simulink model "HRXDUAL_Delay"  (R2023b)
settings: Solver=FixedStepDiscrete  StartTime=0.0  StopTime=Inf  FixedStep=0.0001  RelTol=1e-3  EnableMultiTasking=on
libraries: canmsglib x24, c280xlib x24, simulink x11
(part 1 of 2)
settings Model: SimulationMode=external  ExtModeTrigDuration=8  Creator=eisaa  LastModifiedBy=pc_ha
settings SolverCC: AlgebraicLoopSolver=TrustRegion
settings OptimizationCC: DefaultUnderspecifiedDataType=single  EnhancedBackFolding=on  PassReuseOutputArgsAs=Individual arguments  MaxStackSize=1024  OptimizeBlockOrder=speed  DifferentSizesBufferReuse=on  OptimizationCustomize=off  DenormalBehavior=FlushToZero  EfficientTunableParamExpr=on
settings DebuggingCC: ParameterTunabilityLossMsg=error  UnconnectedInputMsg=warning  UnconnectedOutputMsg=warning  UnconnectedLineMsg=warning
settings HardwareCC: ProdBitPerChar=16  ProdBitPerInt=16  ProdBitPerPointer=32  ProdBitPerSizeT=32  ProdBitPerPtrDiffT=32  ProdLargestAtomicInteger=Integer  ProdLargestAtomicFloat=None  ProdWordSize=16  ProdLongLongMode=on  ProdHWDeviceType=Texas Instruments->C2000
settings ModelReferenceCC: EnableRefExpFcnMdlSchedulingChecks=on
settings SFSimCC: MATLABDynamicMemAlloc=off
settings RTWCC: Description=Embedded Coder  SystemTargetFile=ert.tlc  HardwareBoard=TI Piccolo F28069M LaunchPad  TemplateMakefile=ert_default_tmf  Toolchain=Texas Instruments Code Composer Studio (C2000)  CodeProfilingSaveOptions=AllData  DLArmComputeVersion=19.05
settings CodeAppCC: ForceParamTrailComments=on  IgnoreCustomStorageClasses=off  OperatorAnnotations=on  SimulinkDataObjDesc=on  SFDataObjDesc=on  InsertBlockDesc=on
settings ERTTargetCC: CodeReplacementLibrary=TI C28x  SupportContinuousTime=on  ExtModeTransport=4  ExtModeStaticAlloc=on  ExtModeAutomaticAllocSize=off  ExtModeStaticAllocSize=10000  ExtModeMexFile=ext_xcp  ExtModeMexArgs='127.0.0.1' 0 17725  ExtModeIntrfLevel=Level2 - Open

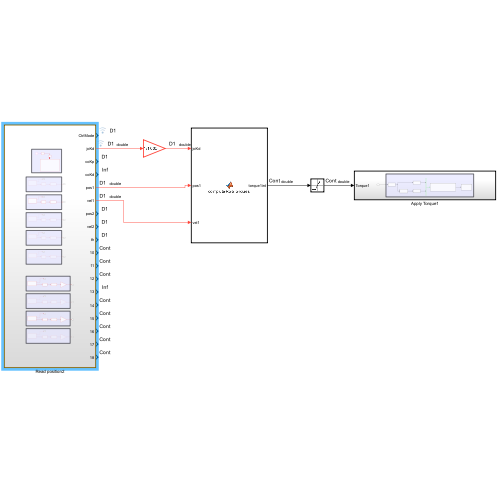
[thumbnail: Simulink's stored preview of the top-level diagram]
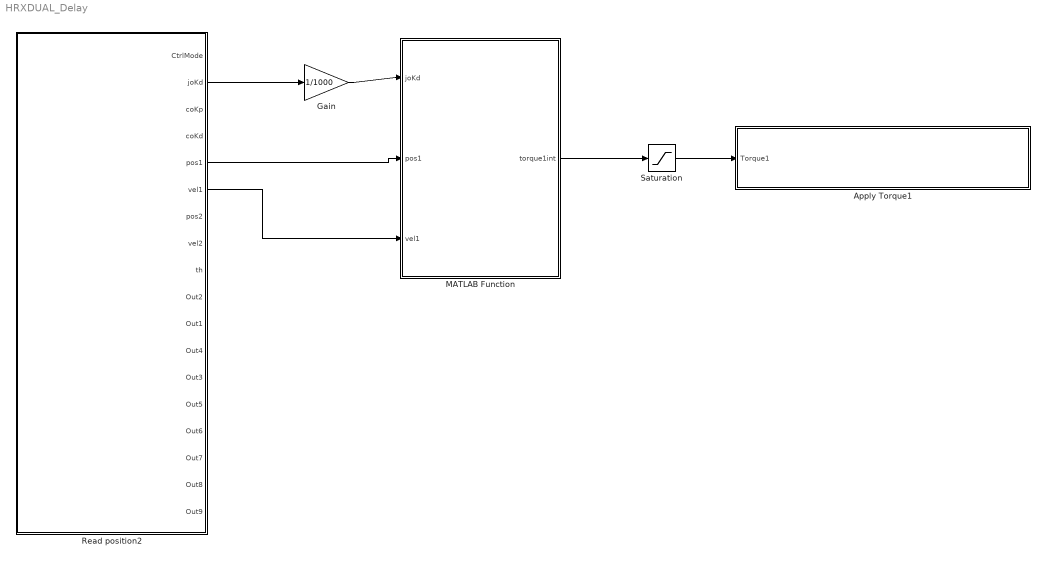
== system HRXDUAL_Delay ==
  Apply Torque1 : Subsystem
  Gain : Gain  Gain=1/1000
  MATLAB Function : MATLAB Function  TreatAsAtomicUnit=on
  Read position2 : Subsystem
  Saturation : Saturate  UpperLimit=1750  LowerLimit=-1750
  wires:
  Read position2/2(joKd) -> Gain/1
  Gain/1 -> MATLAB Function/1(joKd)
  Read position2/5(pos1) -> MATLAB Function/2(pos1)
  Read position2/6(vel1) -> MATLAB Function/3(vel1)
  Saturation/1 -> Apply Torque1/1(Torque1)
  MATLAB Function/1(torque1int) -> Saturation/1

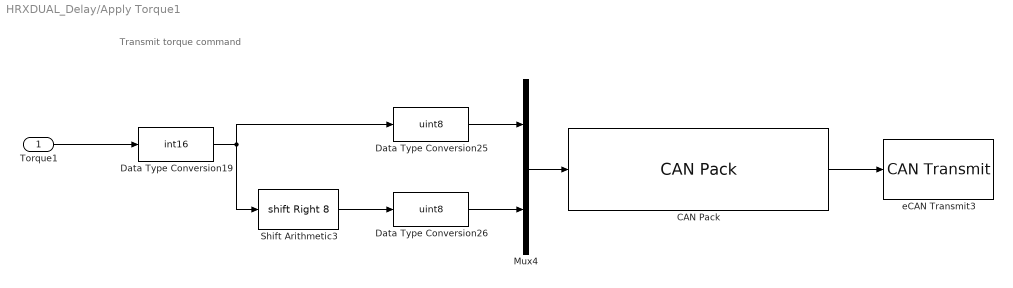
== system HRXDUAL_Delay/Apply Torque1 ==
  note: Transmit torque command
  Torque1 : Inport
  CAN Pack : canmsglib/CAN Pack  MsgList=(none)  MsgName=CAN Msg  MsgIDType=Standard (11-bit identifier)  MsgIdentifier=hex2dec('0x301')  MsgLength=2  Remote=off  ApplyMinMax=off  BusOutput=off  SignalInfo={}
      settings: LibrarySourceBlock=c2000lib/Target Communication/CAN Pack  DataFormat=raw data
  Data Type Conversion19 : DataTypeConversion  OutDataTypeStr=int16  SaturateOnIntegerOverflow=off  RndMeth=Floor
  Data Type Conversion25 : DataTypeConversion  OutDataTypeStr=uint8  SaturateOnIntegerOverflow=off  RndMeth=Floor
  Data Type Conversion26 : DataTypeConversion  OutDataTypeStr=uint8  SaturateOnIntegerOverflow=off  RndMeth=Floor
  Mux4 : Mux  Inputs=2
  Shift Arithmetic3 : ArithShift  BitShiftNumber=8  BitShiftDirection=Right
  eCAN Transmit3 : c280xlib/CAN Transmit  chipFamily=C280x  useModule=CAN_A  mailboxNo=1  messageID=hex2dec('0x301')  messageType=Standard (11-bit identifier)  enableBlockingMode=on  postInterrupt=off  interruptLine=0
  wires:
  CAN Pack/1 -> eCAN Transmit3/1
  Data Type Conversion19/1 -> Data Type Conversion25/1, Shift Arithmetic3/1
  Mux4/1 -> CAN Pack/1
  Data Type Conversion26/1 -> Mux4/2
  Torque1/1 -> Data Type Conversion19/1
  Shift Arithmetic3/1 -> Data Type Conversion26/1
  Data Type Conversion25/1 -> Mux4/1

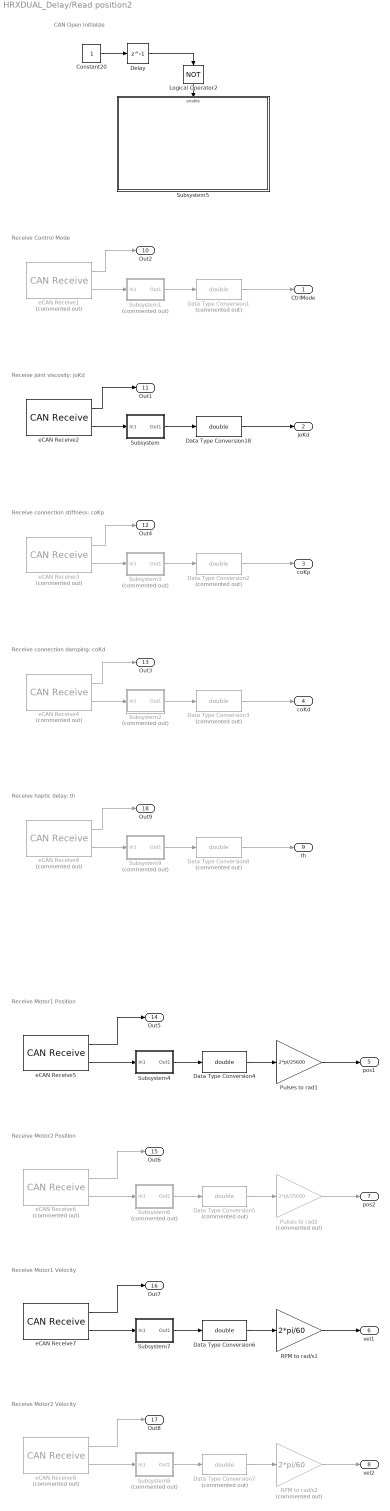
== system HRXDUAL_Delay/Read position2 ==
  note: CAN Open Initialize
  note: Receive Control Mode
  note: Receive joint viscosity: joKd
  note: Receive connection damping: coKd
  note: Receive connection stiffness: coKp
  note: Receive Motor1 Position
  note: Receive Motor2 Position
  note: Receive Motor2 Velocity
  note: Receive Motor1 Velocity
  note: Receive haptic delay: th
  Constant20 : Constant
  Data Type Conversion{1..3,5,7..8} (6 alike) : DataTypeConversion  Commented=on  OutDataTypeStr=double  SaturateOnIntegerOverflow=off  RndMeth=Floor
  Data Type Conversion18 : DataTypeConversion  OutDataTypeStr=double  SaturateOnIntegerOverflow=off  RndMeth=Floor
  Data Type Conversion4 : DataTypeConversion  OutDataTypeStr=double  SaturateOnIntegerOverflow=off  RndMeth=Floor
  Data Type Conversion6 : DataTypeConversion  OutDataTypeStr=double  SaturateOnIntegerOverflow=off  RndMeth=Floor
  Delay : Delay  DelayLength=1
  Logical Operator2 : Logic  Operator=NOT  AllPortsSameDT=off  OutDataTypeStr=boolean
  Pulses to rad1 : Gain  Gain=2*pi/25600
  Pulses to rad2 : Gain  Commented=on  Gain=2*pi/25600
  RPM to rad/s1 : Gain  Gain=2*pi/60
  RPM to rad/s2 : Gain  Commented=on  Gain=2*pi/60
  Subsystem : Subsystem
  Subsystem1 : Subsystem  Commented=on
  Subsystem2 : Subsystem  Commented=on
  Subsystem3 : Subsystem  Commented=on
  Subsystem4 : Subsystem
  Subsystem5 : Subsystem
  Subsystem6 : Subsystem  Commented=on
  Subsystem7 : Subsystem
  Subsystem8 : Subsystem  Commented=on
  Subsystem9 : Subsystem  Commented=on
  eCAN Receive1 : c280xlib/CAN Receive  Commented=on  chipFamily=C280x  useModule=CAN_A  mailboxNo=7  messageID=hex2dec('0x666')  messageType=Standard (11-bit identifier)  enableAcceptanceFiltering=off  messageIDMask=0  sampleTime=-1  dataType=CAN_MESSAGE_TYPE  outputAction=Output last received values  initValue=1  outputMessageID=off  outputMessageLength=off  outputMessageTimeStamp=off  postInterrupt=off  interruptLine=0
  eCAN Receive2 : c280xlib/CAN Receive  chipFamily=C280x  useModule=CAN_A  mailboxNo=8  messageID=hex2dec('0x667')  messageType=Standard (11-bit identifier)  enableAcceptanceFiltering=off  messageIDMask=0  sampleTime=-1  dataType=CAN_MESSAGE_TYPE  outputAction=Output last received values  initValue=0  outputMessageID=off  outputMessageLength=off  outputMessageTimeStamp=off  postInterrupt=off  interruptLine=0
  eCAN Receive3 : c280xlib/CAN Receive  Commented=on  chipFamily=C280x  useModule=CAN_A  mailboxNo=9  messageID=hex2dec('0x668')  messageType=Standard (11-bit identifier)  enableAcceptanceFiltering=off  messageIDMask=0  sampleTime=-1  dataType=CAN_MESSAGE_TYPE  outputAction=Output last received values  initValue=0  outputMessageID=off  outputMessageLength=off  outputMessageTimeStamp=off  postInterrupt=off  interruptLine=0
  eCAN Receive4 : c280xlib/CAN Receive  Commented=on  chipFamily=C280x  useModule=CAN_A  mailboxNo=10  messageID=hex2dec('0x669')  messageType=Standard (11-bit identifier)  enableAcceptanceFiltering=off  messageIDMask=0  sampleTime=-1  dataType=CAN_MESSAGE_TYPE  outputAction=Output last received values  initValue=0  outputMessageID=off  outputMessageLength=off  outputMessageTimeStamp=off  postInterrupt=off  interruptLine=0
  eCAN Receive5 : c280xlib/CAN Receive  chipFamily=C280x  useModule=CAN_A  mailboxNo=3  messageID=hex2dec('0x381')  messageType=Standard (11-bit identifier)  enableAcceptanceFiltering=off  messageIDMask=0  sampleTime=-1  dataType=CAN_MESSAGE_TYPE  outputAction=Output last received values  initValue=0  outputMessageID=off  outputMessageLength=off  outputMessageTimeStamp=off  postInterrupt=off  interruptLine=0
  eCAN Receive6 : c280xlib/CAN Receive  Commented=on  chipFamily=C280x  useModule=CAN_A  mailboxNo=4  messageID=hex2dec('0x382')  messageType=Standard (11-bit identifier)  enableAcceptanceFiltering=off  messageIDMask=0  sampleTime=-1  dataType=CAN_MESSAGE_TYPE  outputAction=Output last received values  initValue=0  outputMessageID=off  outputMessageLength=off  outputMessageTimeStamp=off  postInterrupt=off  interruptLine=0
  eCAN Receive7 : c280xlib/CAN Receive  chipFamily=C280x  useModule=CAN_A  mailboxNo=5  messageID=hex2dec('0x481')  messageType=Standard (11-bit identifier)  enableAcceptanceFiltering=off  messageIDMask=0  sampleTime=-1  dataType=CAN_MESSAGE_TYPE  outputAction=Output last received values  initValue=0  outputMessageID=off  outputMessageLength=off  outputMessageTimeStamp=off  postInterrupt=off  interruptLine=0
  eCAN Receive8 : c280xlib/CAN Receive  Commented=on  chipFamily=C280x  useModule=CAN_A  mailboxNo=6  messageID=hex2dec('0x482')  messageType=Standard (11-bit identifier)  enableAcceptanceFiltering=off  messageIDMask=0  sampleTime=-1  dataType=CAN_MESSAGE_TYPE  outputAction=Output last received values  initValue=0  outputMessageID=off  outputMessageLength=off  outputMessageTimeStamp=off  postInterrupt=off  interruptLine=0
  eCAN Receive9 : c280xlib/CAN Receive  Commented=on  chipFamily=C280x  useModule=CAN_A  mailboxNo=11  messageID=hex2dec('0x66A')  messageType=Standard (11-bit identifier)  enableAcceptanceFiltering=off  messageIDMask=0  sampleTime=-1  dataType=CAN_MESSAGE_TYPE  outputAction=Output last received values  initValue=0  outputMessageID=off  outputMessageLength=off  outputMessageTimeStamp=off  postInterrupt=off  interruptLine=0
  CtrlMode : Outport
  joKd : Outport  Port=2
  coKp : Outport  Port=3
  coKd : Outport  Port=4
  pos1 : Outport  Port=5
  vel1 : Outport  Port=6
  pos2 : Outport  Port=7
  vel2 : Outport  Port=8
  th : Outport  Port=9
  Out2 : Outport  Port=10
  Out1 : Outport  Port=11
  Out4 : Outport  Port=12
  Out3 : Outport  Port=13
  Out5 : Outport  Port=14
  Out6 : Outport  Port=15
  Out7 : Outport  Port=16
  Out8 : Outport  Port=17
  Out9 : Outport  Port=18
  wires:
  Constant20/1 -> Delay/1
  Subsystem/1(Out1) -> Data Type Conversion18/1
  Delay/1 -> Logical Operator2/1
  eCAN Receive2/2 -> Subsystem/1(In1)
  Logical Operator2/1 -> Subsystem5/Enable
  eCAN Receive2/1 -> Out1/1
  Data Type Conversion18/1 -> joKd/1
  eCAN Receive1/2 -> Subsystem1/1(In1)
  Subsystem1/1(Out1) -> Data Type Conversion1/1
  Data Type Conversion1/1 -> CtrlMode/1
  eCAN Receive1/1 -> Out2/1
  eCAN Receive4/1 -> Out3/1
  eCAN Receive3/2 -> Subsystem3/1(In1)
  Subsystem2/1(Out1) -> Data Type Conversion3/1
  Data Type Conversion2/1 -> coKp/1
  eCAN Receive4/2 -> Subsystem2/1(In1)
  Subsystem3/1(Out1) -> Data Type Conversion2/1
  eCAN Receive3/1 -> Out4/1
  Data Type Conversion3/1 -> coKd/1
  eCAN Receive5/1 -> Out5/1
  eCAN Receive5/2 -> Subsystem4/1(In1)
  Subsystem4/1(Out1) -> Data Type Conversion4/1
  Pulses to rad1/1 -> pos1/1
  Data Type Conversion4/1 -> Pulses to rad1/1
  Data Type Conversion5/1 -> Pulses to rad2/1
  Subsystem6/1(Out1) -> Data Type Conversion5/1
  Pulses to rad2/1 -> pos2/1
  eCAN Receive6/2 -> Subsystem6/1(In1)
  eCAN Receive6/1 -> Out6/1
  eCAN Receive8/1 -> Out8/1
  RPM to rad/s2/1 -> vel2/1
  Subsystem8/1(Out1) -> Data Type Conversion7/1
  Data Type Conversion7/1 -> RPM to rad/s2/1
  Data Type Conversion6/1 -> RPM to rad/s1/1
  Subsystem7/1(Out1) -> Data Type Conversion6/1
  RPM to rad/s1/1 -> vel1/1
  eCAN Receive7/2 -> Subsystem7/1(In1)
  eCAN Receive7/1 -> Out7/1
  eCAN Receive8/2 -> Subsystem8/1(In1)
  Data Type Conversion8/1 -> th/1
  eCAN Receive9/2 -> Subsystem9/1(In1)
  Subsystem9/1(Out1) -> Data Type Conversion8/1
  eCAN Receive9/1 -> Out9/1

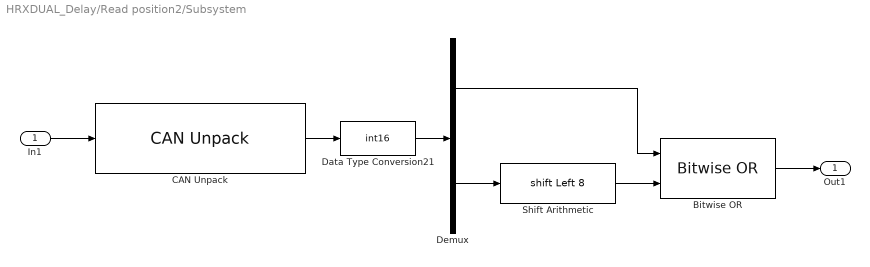
== system HRXDUAL_Delay/Read position2/Subsystem ==
  In1 : Inport
  Bitwise OR : simulink/Logic and Bit Operations/Bitwise Operator  logicop=OR  UseBitMask=off  NumInputPorts=2  BitMask=bin2dec('11011001')  BitMaskRealWorld=Stored Integer
      settings: LibrarySourceBlock=|
      | simulink/Quick Insert/Logic and Bit
      | Operations/Bitwise OR
  CAN Unpack : canmsglib/CAN Unpack  MsgList=(none)  MsgName=CAN Msg  MsgIDType=Standard (11-bit identifier)  MsgIdentifier=-1  MsgLength=2  SignalInfo={}  IDPort=off  TimestampPort=off  ErrorPort=off  RemotePort=off  LengthPort=off  StatusPort=off  ApplyMinMax=off
      settings: LibrarySourceBlock=c2000lib/Target Communication/CAN Unpack  DataFormat=raw data
  Data Type Conversion21 : DataTypeConversion  OutDataTypeStr=int16  SaturateOnIntegerOverflow=off  RndMeth=Floor
  Demux : Demux  Outputs=2
  Shift Arithmetic : ArithShift  BitShiftNumber=8  BitShiftDirection=Left
  Out1 : Outport
  wires:
  Shift Arithmetic/1 -> Bitwise OR/2
  Demux/2 -> Shift Arithmetic/1
  CAN Unpack/1 -> Data Type Conversion21/1
  Demux/1 -> Bitwise OR/1
  Data Type Conversion21/1 -> Demux/1
  Bitwise OR/1 -> Out1/1
  In1/1 -> CAN Unpack/1

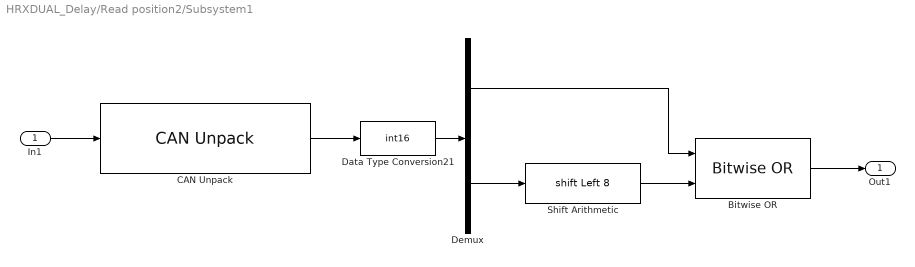
== system HRXDUAL_Delay/Read position2/Subsystem1 ==
  In1 : Inport
  Bitwise OR : simulink/Logic and Bit Operations/Bitwise Operator  logicop=OR  UseBitMask=off  NumInputPorts=2  BitMask=bin2dec('11011001')  BitMaskRealWorld=Stored Integer
      settings: LibrarySourceBlock=|
      | simulink/Quick Insert/Logic and Bit
      | Operations/Bitwise OR
  CAN Unpack : canmsglib/CAN Unpack  MsgList=(none)  MsgName=CAN Msg  MsgIDType=Standard (11-bit identifier)  MsgIdentifier=-1  MsgLength=2  SignalInfo={}  IDPort=off  TimestampPort=off  ErrorPort=off  RemotePort=off  LengthPort=off  StatusPort=off  ApplyMinMax=off
      settings: LibrarySourceBlock=c2000lib/Target Communication/CAN Unpack  DataFormat=raw data
  Data Type Conversion21 : DataTypeConversion  OutDataTypeStr=int16  SaturateOnIntegerOverflow=off  RndMeth=Floor
  Demux : Demux  Outputs=2
  Shift Arithmetic : ArithShift  BitShiftNumber=8  BitShiftDirection=Left
  Out1 : Outport
  wires:
  Shift Arithmetic/1 -> Bitwise OR/2
  Demux/2 -> Shift Arithmetic/1
  CAN Unpack/1 -> Data Type Conversion21/1
  Demux/1 -> Bitwise OR/1
  Data Type Conversion21/1 -> Demux/1
  Bitwise OR/1 -> Out1/1
  In1/1 -> CAN Unpack/1

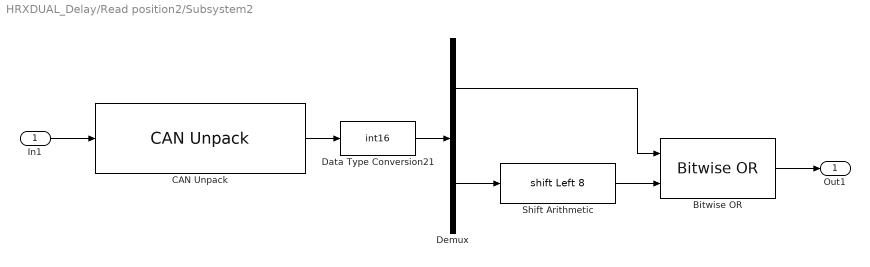
== system HRXDUAL_Delay/Read position2/Subsystem2 ==
  In1 : Inport
  Bitwise OR : simulink/Logic and Bit Operations/Bitwise Operator  logicop=OR  UseBitMask=off  NumInputPorts=2  BitMask=bin2dec('11011001')  BitMaskRealWorld=Stored Integer
      settings: LibrarySourceBlock=|
      | simulink/Quick Insert/Logic and Bit
      | Operations/Bitwise OR
  CAN Unpack : canmsglib/CAN Unpack  MsgList=(none)  MsgName=CAN Msg  MsgIDType=Standard (11-bit identifier)  MsgIdentifier=-1  MsgLength=2  SignalInfo={}  IDPort=off  TimestampPort=off  ErrorPort=off  RemotePort=off  LengthPort=off  StatusPort=off  ApplyMinMax=off
      settings: LibrarySourceBlock=c2000lib/Target Communication/CAN Unpack  DataFormat=raw data
  Data Type Conversion21 : DataTypeConversion  OutDataTypeStr=int16  SaturateOnIntegerOverflow=off  RndMeth=Floor
  Demux : Demux  Outputs=2
  Shift Arithmetic : ArithShift  BitShiftNumber=8  BitShiftDirection=Left
  Out1 : Outport
  wires:
  Shift Arithmetic/1 -> Bitwise OR/2
  Demux/2 -> Shift Arithmetic/1
  CAN Unpack/1 -> Data Type Conversion21/1
  Demux/1 -> Bitwise OR/1
  Data Type Conversion21/1 -> Demux/1
  Bitwise OR/1 -> Out1/1
  In1/1 -> CAN Unpack/1

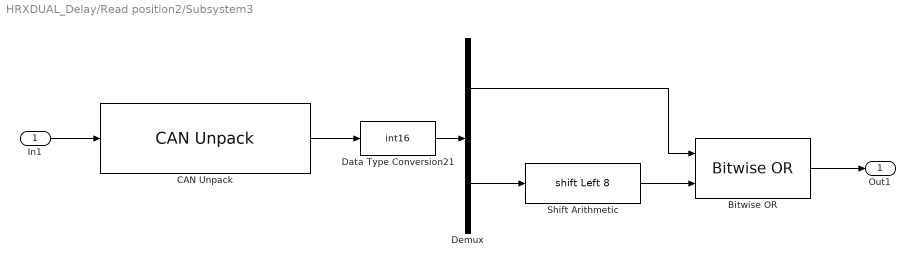
== system HRXDUAL_Delay/Read position2/Subsystem3 ==
  In1 : Inport
  Bitwise OR : simulink/Logic and Bit Operations/Bitwise Operator  logicop=OR  UseBitMask=off  NumInputPorts=2  BitMask=bin2dec('11011001')  BitMaskRealWorld=Stored Integer
      settings: LibrarySourceBlock=|
      | simulink/Quick Insert/Logic and Bit
      | Operations/Bitwise OR
  CAN Unpack : canmsglib/CAN Unpack  MsgList=(none)  MsgName=CAN Msg  MsgIDType=Standard (11-bit identifier)  MsgIdentifier=-1  MsgLength=2  SignalInfo={}  IDPort=off  TimestampPort=off  ErrorPort=off  RemotePort=off  LengthPort=off  StatusPort=off  ApplyMinMax=off
      settings: LibrarySourceBlock=c2000lib/Target Communication/CAN Unpack  DataFormat=raw data
  Data Type Conversion21 : DataTypeConversion  OutDataTypeStr=int16  SaturateOnIntegerOverflow=off  RndMeth=Floor
  Demux : Demux  Outputs=2
  Shift Arithmetic : ArithShift  BitShiftNumber=8  BitShiftDirection=Left
  Out1 : Outport
  wires:
  Shift Arithmetic/1 -> Bitwise OR/2
  Demux/2 -> Shift Arithmetic/1
  CAN Unpack/1 -> Data Type Conversion21/1
  Demux/1 -> Bitwise OR/1
  Data Type Conversion21/1 -> Demux/1
  Bitwise OR/1 -> Out1/1
  In1/1 -> CAN Unpack/1

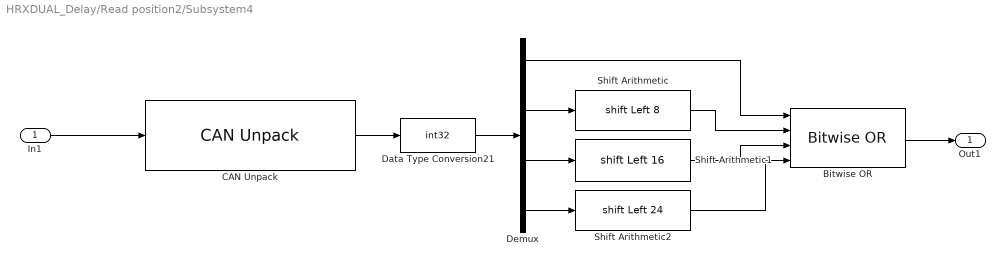
== system HRXDUAL_Delay/Read position2/Subsystem4 ==
  In1 : Inport
  Bitwise OR : simulink/Logic and Bit Operations/Bitwise Operator  logicop=OR  UseBitMask=off  NumInputPorts=4  BitMask=bin2dec('11011001')  BitMaskRealWorld=Stored Integer
      settings: LibrarySourceBlock=|
      | simulink/Quick Insert/Logic and Bit
      | Operations/Bitwise OR
  CAN Unpack : canmsglib/CAN Unpack  MsgList=(none)  MsgName=CAN Msg  MsgIDType=Standard (11-bit identifier)  MsgIdentifier=-1  MsgLength=4  SignalInfo={}  IDPort=off  TimestampPort=off  ErrorPort=off  RemotePort=off  LengthPort=off  StatusPort=off  ApplyMinMax=off
      settings: LibrarySourceBlock=c2000lib/Target Communication/CAN Unpack  DataFormat=raw data
  Data Type Conversion21 : DataTypeConversion  OutDataTypeStr=int32  SaturateOnIntegerOverflow=off  RndMeth=Floor
  Demux : Demux
  Shift Arithmetic : ArithShift  BitShiftNumber=8  BitShiftDirection=Left
  Shift Arithmetic1 : ArithShift  BitShiftNumber=16  BitShiftDirection=Left
  Shift Arithmetic2 : ArithShift  BitShiftNumber=24  BitShiftDirection=Left
  Out1 : Outport
  wires:
  Shift Arithmetic/1 -> Bitwise OR/2
  Shift Arithmetic2/1 -> Bitwise OR/4
  Demux/2 -> Shift Arithmetic/1
  Demux/3 -> Shift Arithmetic1/1
  Shift Arithmetic1/1 -> Bitwise OR/3
  Demux/4 -> Shift Arithmetic2/1
  CAN Unpack/1 -> Data Type Conversion21/1
  Demux/1 -> Bitwise OR/1
  Data Type Conversion21/1 -> Demux/1
  Bitwise OR/1 -> Out1/1
  In1/1 -> CAN Unpack/1

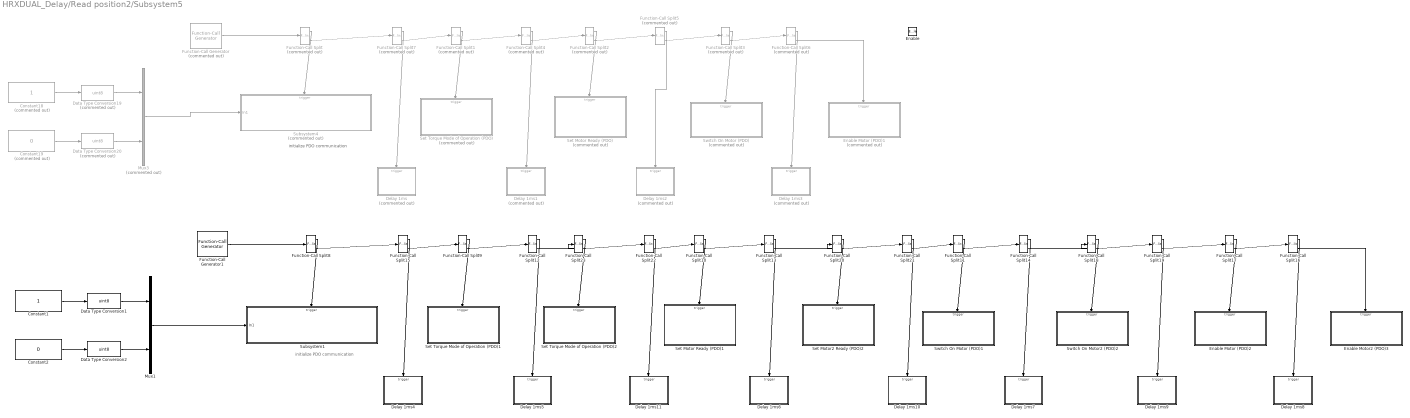
== system HRXDUAL_Delay/Read position2/Subsystem5 ==
  note: initialize PDO communication
  note: initialize PDO communication
  Enable : EnablePort
  Constant1 : Constant
  Constant18 : Constant  Commented=on
  Constant19 : Constant  Commented=on  Value=0
  Constant2 : Constant  Value=0
  Data Type Conversion1 : DataTypeConversion  OutDataTypeStr=uint8  SaturateOnIntegerOverflow=off  RndMeth=Floor
  Data Type Conversion19 : DataTypeConversion  Commented=on  OutDataTypeStr=uint8  SaturateOnIntegerOverflow=off  RndMeth=Floor
  Data Type Conversion2 : DataTypeConversion  OutDataTypeStr=uint8  SaturateOnIntegerOverflow=off  RndMeth=Floor
  Data Type Conversion20 : DataTypeConversion  Commented=on  OutDataTypeStr=uint8  SaturateOnIntegerOverflow=off  RndMeth=Floor
  Delay 1ms : Subsystem  Commented=on  TreatAsAtomicUnit=on
  Delay 1ms1 : Subsystem  Commented=on  TreatAsAtomicUnit=on
  Delay 1ms10 : Subsystem  TreatAsAtomicUnit=on
  Delay 1ms11 : Subsystem  TreatAsAtomicUnit=on
  Delay 1ms2 : Subsystem  Commented=on  TreatAsAtomicUnit=on
  Delay 1ms3 : Subsystem  Commented=on  TreatAsAtomicUnit=on
  Delay 1ms4 : Subsystem  TreatAsAtomicUnit=on
  Delay 1ms5 : Subsystem  TreatAsAtomicUnit=on
  Delay 1ms6 : Subsystem  TreatAsAtomicUnit=on
  Delay 1ms7 : Subsystem  TreatAsAtomicUnit=on
  Delay 1ms8 : Subsystem  TreatAsAtomicUnit=on
  Delay 1ms9 : Subsystem  TreatAsAtomicUnit=on
  Enable Motor (PDO)1 : Subsystem  Commented=on
  Enable Motor (PDO)2 : Subsystem
  Enable Motor2 (PDO)3 : Subsystem
  Function-Call Generator : simulink/Ports & Subsystems/Function-Call Generator  Commented=on  sample_time=-1  numberOfIterations=1  DisallowWideOutput=off
  Function-Call Generator1 : simulink/Ports & Subsystems/Function-Call Generator  sample_time=-1  numberOfIterations=1  DisallowWideOutput=off
  Function-Call Split{,1..7} (8 alike) : FunctionCallSplit  Commented=on  NumOutputPorts=2
  Function-Call Split{8..23} (16 alike) : FunctionCallSplit  NumOutputPorts=2
  Mux1 : Mux  Inputs=2
  Mux3 : Mux  Commented=on  Inputs=2
  Set Motor Ready (PDO) : Subsystem  Commented=on
  Set Motor Ready (PDO)1 : Subsystem
  Set Motor2 Ready (PDO)2 : Subsystem
  Set Torque Mode of Operation (PDO) : Subsystem  Commented=on
  Set Torque Mode of Operation (PDO)1 : Subsystem
  Set Torque Mode of Operation (PDO)2 : Subsystem
  Subsystem1 : Subsystem
  Subsystem4 : Subsystem  Commented=on
  Switch On Motor (PDO) : Subsystem  Commented=on
  Switch On Motor (PDO)1 : Subsystem
  Switch On Motor2 (PDO)2 : Subsystem
  wires:
  Function-Call Split2/1 -> Set Motor Ready (PDO)/Trigger
  Function-Call Split6/2 -> Enable Motor (PDO)1/Trigger
  Data Type Conversion20/1 -> Mux3/2
  Data Type Conversion19/1 -> Mux3/1
  Function-Call Split/2 -> Function-Call Split7/1
  Function-Call Split5/2 -> Function-Call Split3/1
  Function-Call Split6/1 -> Delay 1ms3/Trigger
  Function-Call Split1/1 -> Set Torque Mode of Operation (PDO)/Trigger
  Function-Call Generator/1 -> Function-Call Split/1
  Mux3/1 -> Subsystem4/1(In1)
  Function-Call Split7/2 -> Function-Call Split1/1
  Function-Call Split/1 -> Subsystem4/Trigger
  Constant19/1 -> Data Type Conversion20/1
  Function-Call Split4/1 -> Delay 1ms1/Trigger
  Constant18/1 -> Data Type Conversion19/1
  Function-Call Split2/2 -> Function-Call Split5/1
  Function-Call Split5/1 -> Delay 1ms2/Trigger
  Function-Call Split1/2 -> Function-Call Split4/1
  Function-Call Split7/1 -> Delay 1ms/Trigger
  Function-Call Split3/1 -> Switch On Motor (PDO)/Trigger
  Function-Call Split4/2 -> Function-Call Split2/1
  Function-Call Split3/2 -> Function-Call Split6/1
  Constant2/1 -> Data Type Conversion2/1
  Constant1/1 -> Data Type Conversion1/1
  Function-Call Split11/1 -> Switch On Motor (PDO)1/Trigger
  Function-Call Generator1/1 -> Function-Call Split8/1
  Function-Call Split9/1 -> Set Torque Mode of Operation (PDO)1/Trigger
  Function-Call Split11/2 -> Function-Call Split14/1
  Function-Call Split8/1 -> Subsystem1/Trigger
  Function-Call Split15/1 -> Delay 1ms4/Trigger
  Function-Call Split9/2 -> Function-Call Split12/1
  Function-Call Split10/2 -> Function-Call Split13/1
  Function-Call Split13/1 -> Delay 1ms6/Trigger
  Data Type Conversion2/1 -> Mux1/2
  Function-Call Split12/1 -> Delay 1ms5/Trigger
  Function-Call Split14/1 -> Delay 1ms7/Trigger
  Mux1/1 -> Subsystem1/1(In1)
  Data Type Conversion1/1 -> Mux1/1
  Function-Call Split15/2 -> Function-Call Split9/1
  Function-Call Split10/1 -> Set Motor Ready (PDO)1/Trigger
  Function-Call Split21/2 -> Function-Call Split11/1
  Function-Call Split8/2 -> Function-Call Split15/1
  Function-Call Split16/2 -> Enable Motor2 (PDO)3/Trigger
  Function-Call Split16/1 -> Delay 1ms8/Trigger
  Function-Call Split17/1 -> Enable Motor (PDO)2/Trigger
  Function-Call Split17/2 -> Function-Call Split16/1
  Function-Call Split19/2 -> Function-Call Split17/1
  Function-Call Split19/1 -> Delay 1ms9/Trigger
  Function-Call Split14/2 -> Function-Call Split18/1
  Function-Call Split18/1 -> Switch On Motor2 (PDO)2/Trigger
  Function-Call Split18/2 -> Function-Call Split19/1
  Function-Call Split21/1 -> Delay 1ms10/Trigger
  Function-Call Split20/2 -> Function-Call Split21/1
  Function-Call Split13/2 -> Function-Call Split20/1
  Function-Call Split20/1 -> Set Motor2 Ready (PDO)2/Trigger
  Function-Call Split12/2 -> Function-Call Split23/1
  Function-Call Split22/1 -> Delay 1ms11/Trigger
  Function-Call Split23/2 -> Function-Call Split22/1
  Function-Call Split23/1 -> Set Torque Mode of Operation (PDO)2/Trigger
  Function-Call Split22/2 -> Function-Call Split10/1

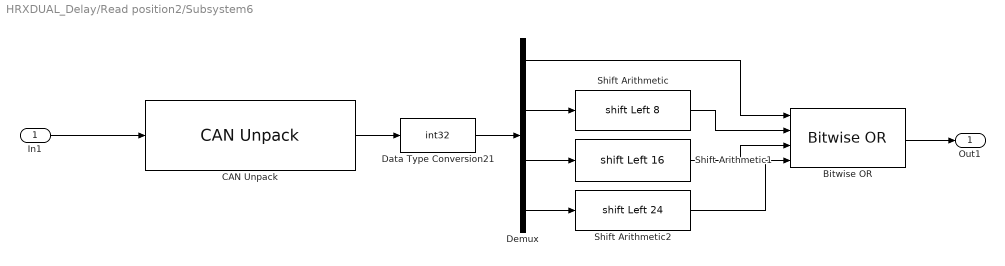
== system HRXDUAL_Delay/Read position2/Subsystem6 ==
  In1 : Inport
  Bitwise OR : simulink/Logic and Bit Operations/Bitwise Operator  logicop=OR  UseBitMask=off  NumInputPorts=4  BitMask=bin2dec('11011001')  BitMaskRealWorld=Stored Integer
      settings: LibrarySourceBlock=|
      | simulink/Quick Insert/Logic and Bit
      | Operations/Bitwise OR
  CAN Unpack : canmsglib/CAN Unpack  MsgList=(none)  MsgName=CAN Msg  MsgIDType=Standard (11-bit identifier)  MsgIdentifier=-1  MsgLength=4  SignalInfo={}  IDPort=off  TimestampPort=off  ErrorPort=off  RemotePort=off  LengthPort=off  StatusPort=off  ApplyMinMax=off
      settings: LibrarySourceBlock=c2000lib/Target Communication/CAN Unpack  DataFormat=raw data
  Data Type Conversion21 : DataTypeConversion  OutDataTypeStr=int32  SaturateOnIntegerOverflow=off  RndMeth=Floor
  Demux : Demux
  Shift Arithmetic : ArithShift  BitShiftNumber=8  BitShiftDirection=Left
  Shift Arithmetic1 : ArithShift  BitShiftNumber=16  BitShiftDirection=Left
  Shift Arithmetic2 : ArithShift  BitShiftNumber=24  BitShiftDirection=Left
  Out1 : Outport
  wires:
  Shift Arithmetic/1 -> Bitwise OR/2
  Shift Arithmetic2/1 -> Bitwise OR/4
  Demux/2 -> Shift Arithmetic/1
  Demux/3 -> Shift Arithmetic1/1
  Shift Arithmetic1/1 -> Bitwise OR/3
  Demux/4 -> Shift Arithmetic2/1
  CAN Unpack/1 -> Data Type Conversion21/1
  Demux/1 -> Bitwise OR/1
  Data Type Conversion21/1 -> Demux/1
  Bitwise OR/1 -> Out1/1
  In1/1 -> CAN Unpack/1

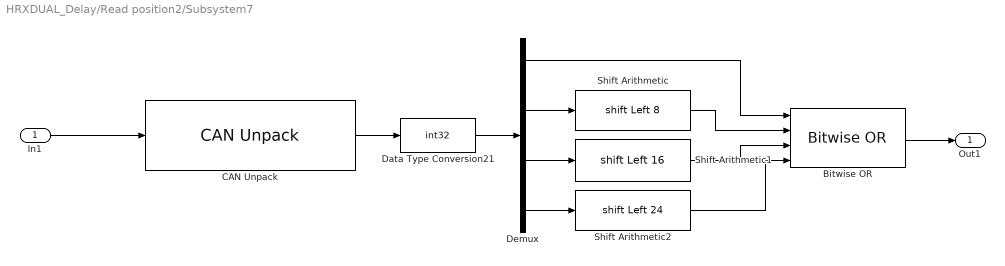
== system HRXDUAL_Delay/Read position2/Subsystem7 ==
  In1 : Inport
  Bitwise OR : simulink/Logic and Bit Operations/Bitwise Operator  logicop=OR  UseBitMask=off  NumInputPorts=4  BitMask=bin2dec('11011001')  BitMaskRealWorld=Stored Integer
      settings: LibrarySourceBlock=|
      | simulink/Quick Insert/Logic and Bit
      | Operations/Bitwise OR
  CAN Unpack : canmsglib/CAN Unpack  MsgList=(none)  MsgName=CAN Msg  MsgIDType=Standard (11-bit identifier)  MsgIdentifier=-1  MsgLength=4  SignalInfo={}  IDPort=off  TimestampPort=off  ErrorPort=off  RemotePort=off  LengthPort=off  StatusPort=off  ApplyMinMax=off
      settings: LibrarySourceBlock=c2000lib/Target Communication/CAN Unpack  DataFormat=raw data
  Data Type Conversion21 : DataTypeConversion  OutDataTypeStr=int32  SaturateOnIntegerOverflow=off  RndMeth=Floor
  Demux : Demux
  Shift Arithmetic : ArithShift  BitShiftNumber=8  BitShiftDirection=Left
  Shift Arithmetic1 : ArithShift  BitShiftNumber=16  BitShiftDirection=Left
  Shift Arithmetic2 : ArithShift  BitShiftNumber=24  BitShiftDirection=Left
  Out1 : Outport
  wires:
  Shift Arithmetic/1 -> Bitwise OR/2
  Shift Arithmetic2/1 -> Bitwise OR/4
  Demux/2 -> Shift Arithmetic/1
  Demux/3 -> Shift Arithmetic1/1
  Shift Arithmetic1/1 -> Bitwise OR/3
  Demux/4 -> Shift Arithmetic2/1
  CAN Unpack/1 -> Data Type Conversion21/1
  Demux/1 -> Bitwise OR/1
  Data Type Conversion21/1 -> Demux/1
  Bitwise OR/1 -> Out1/1
  In1/1 -> CAN Unpack/1

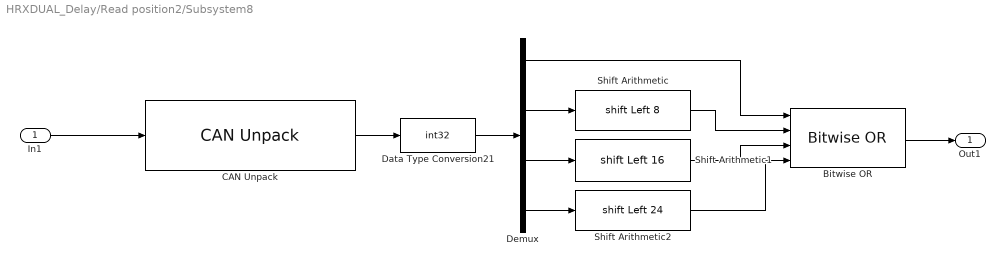
== system HRXDUAL_Delay/Read position2/Subsystem8 ==
  In1 : Inport
  Bitwise OR : simulink/Logic and Bit Operations/Bitwise Operator  logicop=OR  UseBitMask=off  NumInputPorts=4  BitMask=bin2dec('11011001')  BitMaskRealWorld=Stored Integer
      settings: LibrarySourceBlock=|
      | simulink/Quick Insert/Logic and Bit
      | Operations/Bitwise OR
  CAN Unpack : canmsglib/CAN Unpack  MsgList=(none)  MsgName=CAN Msg  MsgIDType=Standard (11-bit identifier)  MsgIdentifier=-1  MsgLength=4  SignalInfo={}  IDPort=off  TimestampPort=off  ErrorPort=off  RemotePort=off  LengthPort=off  StatusPort=off  ApplyMinMax=off
      settings: LibrarySourceBlock=c2000lib/Target Communication/CAN Unpack  DataFormat=raw data
  Data Type Conversion21 : DataTypeConversion  OutDataTypeStr=int32  SaturateOnIntegerOverflow=off  RndMeth=Floor
  Demux : Demux
  Shift Arithmetic : ArithShift  BitShiftNumber=8  BitShiftDirection=Left
  Shift Arithmetic1 : ArithShift  BitShiftNumber=16  BitShiftDirection=Left
  Shift Arithmetic2 : ArithShift  BitShiftNumber=24  BitShiftDirection=Left
  Out1 : Outport
  wires:
  Shift Arithmetic/1 -> Bitwise OR/2
  Shift Arithmetic2/1 -> Bitwise OR/4
  Demux/2 -> Shift Arithmetic/1
  Demux/3 -> Shift Arithmetic1/1
  Shift Arithmetic1/1 -> Bitwise OR/3
  Demux/4 -> Shift Arithmetic2/1
  CAN Unpack/1 -> Data Type Conversion21/1
  Demux/1 -> Bitwise OR/1
  Data Type Conversion21/1 -> Demux/1
  Bitwise OR/1 -> Out1/1
  In1/1 -> CAN Unpack/1

== system HRXDUAL_Delay/Read position2/Subsystem9 ==
  In1 : Inport
  Bitwise OR : simulink/Logic and Bit Operations/Bitwise Operator  logicop=OR  UseBitMask=off  NumInputPorts=2  BitMask=bin2dec('11011001')  BitMaskRealWorld=Stored Integer
      settings: LibrarySourceBlock=|
      | simulink/Quick Insert/Logic and Bit
      | Operations/Bitwise OR
  CAN Unpack : canmsglib/CAN Unpack  MsgList=(none)  MsgName=CAN Msg  MsgIDType=Standard (11-bit identifier)  MsgIdentifier=-1  MsgLength=2  SignalInfo={}  IDPort=off  TimestampPort=off  ErrorPort=off  RemotePort=off  LengthPort=off  StatusPort=off  ApplyMinMax=off
      settings: LibrarySourceBlock=c2000lib/Target Communication/CAN Unpack  DataFormat=raw data
  Data Type Conversion21 : DataTypeConversion  OutDataTypeStr=int16  SaturateOnIntegerOverflow=off  RndMeth=Floor
  Demux : Demux  Outputs=2
  Shift Arithmetic : ArithShift  BitShiftNumber=8  BitShiftDirection=Left
  Out1 : Outport
  wires:
  In1/1 -> CAN Unpack/1
  Bitwise OR/1 -> Out1/1
  Data Type Conversion21/1 -> Demux/1
  Demux/1 -> Bitwise OR/1
  CAN Unpack/1 -> Data Type Conversion21/1
  Demux/2 -> Shift Arithmetic/1
  Shift Arithmetic/1 -> Bitwise OR/2

== system HRXDUAL_Delay/Read position2/Subsystem5/Delay 1ms ==
  function : TriggerPort  TriggerType=function-call  VariantControl=Variant
  System Outputs : Subsystem  mask(System Outputs){ShowInLibBrowser=0}
      mask prompts: ShowInLibBrowser "Simulink:masks:CustCodeMaskParam1_MP"
      settings: CopyFcn=cccopyfcn(gcb)  OpenFcn=ccopenfcn('System Outputs Function')
      mask Help: eval('feval(''rtwprivate'',''rtwhelpview'',''rtw_sys_outputs_block'')');
      mask Display: disp('System\nOutputs');

== system HRXDUAL_Delay/Read position2/Subsystem5/Delay 1ms1 ==
  function : TriggerPort  TriggerType=function-call  VariantControl=Variant
  System Outputs : Subsystem  mask(System Outputs){ShowInLibBrowser=0}
      mask prompts: ShowInLibBrowser "Simulink:masks:CustCodeMaskParam1_MP"
      settings: CopyFcn=cccopyfcn(gcb)  OpenFcn=ccopenfcn('System Outputs Function')
      mask Help: eval('feval(''rtwprivate'',''rtwhelpview'',''rtw_sys_outputs_block'')');
      mask Display: disp('System\nOutputs');

== system HRXDUAL_Delay/Read position2/Subsystem5/Delay 1ms10 ==
  function : TriggerPort  TriggerType=function-call  VariantControl=Variant
  System Outputs : Subsystem  mask(System Outputs){ShowInLibBrowser=0}
      mask prompts: ShowInLibBrowser "Simulink:masks:CustCodeMaskParam1_MP"
      settings: CopyFcn=cccopyfcn(gcb)  OpenFcn=ccopenfcn('System Outputs Function')
      mask Help: eval('feval(''rtwprivate'',''rtwhelpview'',''rtw_sys_outputs_block'')');
      mask Display: disp('System\nOutputs');

== system HRXDUAL_Delay/Read position2/Subsystem5/Delay 1ms11 ==
  function : TriggerPort  TriggerType=function-call  VariantControl=Variant
  System Outputs : Subsystem  mask(System Outputs){ShowInLibBrowser=0}
      mask prompts: ShowInLibBrowser "Simulink:masks:CustCodeMaskParam1_MP"
      settings: CopyFcn=cccopyfcn(gcb)  OpenFcn=ccopenfcn('System Outputs Function')
      mask Help: eval('feval(''rtwprivate'',''rtwhelpview'',''rtw_sys_outputs_block'')');
      mask Display: disp('System\nOutputs');

== system HRXDUAL_Delay/Read position2/Subsystem5/Delay 1ms2 ==
  function : TriggerPort  TriggerType=function-call  VariantControl=Variant
  System Outputs : Subsystem  mask(System Outputs){ShowInLibBrowser=0}
      mask prompts: ShowInLibBrowser "Simulink:masks:CustCodeMaskParam1_MP"
      settings: CopyFcn=cccopyfcn(gcb)  OpenFcn=ccopenfcn('System Outputs Function')
      mask Help: eval('feval(''rtwprivate'',''rtwhelpview'',''rtw_sys_outputs_block'')');
      mask Display: disp('System\nOutputs');

== system HRXDUAL_Delay/Read position2/Subsystem5/Delay 1ms3 ==
  function : TriggerPort  TriggerType=function-call  VariantControl=Variant
  System Outputs : Subsystem  mask(System Outputs){ShowInLibBrowser=0}
      mask prompts: ShowInLibBrowser "Simulink:masks:CustCodeMaskParam1_MP"
      settings: CopyFcn=cccopyfcn(gcb)  OpenFcn=ccopenfcn('System Outputs Function')
      mask Help: eval('feval(''rtwprivate'',''rtwhelpview'',''rtw_sys_outputs_block'')');
      mask Display: disp('System\nOutputs');

== system HRXDUAL_Delay/Read position2/Subsystem5/Delay 1ms4 ==
  function : TriggerPort  TriggerType=function-call  VariantControl=Variant
  System Outputs : Subsystem  mask(System Outputs){ShowInLibBrowser=0}
      mask prompts: ShowInLibBrowser "Simulink:masks:CustCodeMaskParam1_MP"
      settings: CopyFcn=cccopyfcn(gcb)  OpenFcn=ccopenfcn('System Outputs Function')
      mask Help: eval('feval(''rtwprivate'',''rtwhelpview'',''rtw_sys_outputs_block'')');
      mask Display: disp('System\nOutputs');

== system HRXDUAL_Delay/Read position2/Subsystem5/Delay 1ms5 ==
  function : TriggerPort  TriggerType=function-call  VariantControl=Variant
  System Outputs : Subsystem  mask(System Outputs){ShowInLibBrowser=0}
      mask prompts: ShowInLibBrowser "Simulink:masks:CustCodeMaskParam1_MP"
      settings: CopyFcn=cccopyfcn(gcb)  OpenFcn=ccopenfcn('System Outputs Function')
      mask Help: eval('feval(''rtwprivate'',''rtwhelpview'',''rtw_sys_outputs_block'')');
      mask Display: disp('System\nOutputs');

== system HRXDUAL_Delay/Read position2/Subsystem5/Delay 1ms6 ==
  function : TriggerPort  TriggerType=function-call  VariantControl=Variant
  System Outputs : Subsystem  mask(System Outputs){ShowInLibBrowser=0}
      mask prompts: ShowInLibBrowser "Simulink:masks:CustCodeMaskParam1_MP"
      settings: CopyFcn=cccopyfcn(gcb)  OpenFcn=ccopenfcn('System Outputs Function')
      mask Help: eval('feval(''rtwprivate'',''rtwhelpview'',''rtw_sys_outputs_block'')');
      mask Display: disp('System\nOutputs');

== system HRXDUAL_Delay/Read position2/Subsystem5/Delay 1ms7 ==
  function : TriggerPort  TriggerType=function-call  VariantControl=Variant
  System Outputs : Subsystem  mask(System Outputs){ShowInLibBrowser=0}
      mask prompts: ShowInLibBrowser "Simulink:masks:CustCodeMaskParam1_MP"
      settings: CopyFcn=cccopyfcn(gcb)  OpenFcn=ccopenfcn('System Outputs Function')
      mask Help: eval('feval(''rtwprivate'',''rtwhelpview'',''rtw_sys_outputs_block'')');
      mask Display: disp('System\nOutputs');

== system HRXDUAL_Delay/Read position2/Subsystem5/Delay 1ms8 ==
  function : TriggerPort  TriggerType=function-call  VariantControl=Variant
  System Outputs : Subsystem  mask(System Outputs){ShowInLibBrowser=0}
      mask prompts: ShowInLibBrowser "Simulink:masks:CustCodeMaskParam1_MP"
      settings: CopyFcn=cccopyfcn(gcb)  OpenFcn=ccopenfcn('System Outputs Function')
      mask Help: eval('feval(''rtwprivate'',''rtwhelpview'',''rtw_sys_outputs_block'')');
      mask Display: disp('System\nOutputs');

== system HRXDUAL_Delay/Read position2/Subsystem5/Delay 1ms9 ==
  function : TriggerPort  TriggerType=function-call  VariantControl=Variant
  System Outputs : Subsystem  mask(System Outputs){ShowInLibBrowser=0}
      mask prompts: ShowInLibBrowser "Simulink:masks:CustCodeMaskParam1_MP"
      settings: CopyFcn=cccopyfcn(gcb)  OpenFcn=ccopenfcn('System Outputs Function')
      mask Help: eval('feval(''rtwprivate'',''rtwhelpview'',''rtw_sys_outputs_block'')');
      mask Display: disp('System\nOutputs');

== system HRXDUAL_Delay/Read position2/Subsystem5/Enable Motor (PDO)1 ==
  function : TriggerPort  TriggerType=function-call  VariantControl=(inherit)
  CAN Pack : canmsglib/CAN Pack  MsgList=(none)  MsgName=CAN Msg  MsgIDType=Standard (11-bit identifier)  MsgIdentifier=hex2dec('0x202')  MsgLength=3  Remote=off  ApplyMinMax=off  BusOutput=off  SignalInfo={ 'Signal1', '0', '8', 'BE', 'unsigned', 'Standard', '0', '1', '0', '-Inf', 'Inf' }
      settings: LibrarySourceBlock=c2000lib/Target Communication/CAN Pack  DataFormat=raw data
  Constant22 : Constant  Value=10  OutDataTypeStr=uint8
  Constant23 : Constant  Value=0  OutDataTypeStr=uint8
  Constant24 : Constant  Value=hex2dec('0x0F')  OutDataTypeStr=uint8
  Mux4 : Mux  Inputs=3
  eCAN Transmit3 : c280xlib/CAN Transmit  chipFamily=C280x  useModule=CAN_A  mailboxNo=1  messageID=hex2dec('0x202')  messageType=Standard (11-bit identifier)  enableBlockingMode=on  postInterrupt=off  interruptLine=0
  wires:
  Mux4/1 -> CAN Pack/1
  CAN Pack/1 -> eCAN Transmit3/1
  Constant22/1 -> Mux4/3
  Constant23/1 -> Mux4/2
  Constant24/1 -> Mux4/1

== system HRXDUAL_Delay/Read position2/Subsystem5/Enable Motor (PDO)2 ==
  function : TriggerPort  TriggerType=function-call  VariantControl=(inherit)
  CAN Pack : canmsglib/CAN Pack  MsgList=(none)  MsgName=CAN Msg  MsgIDType=Standard (11-bit identifier)  MsgIdentifier=hex2dec('0x201')  MsgLength=3  Remote=off  ApplyMinMax=off  BusOutput=off  SignalInfo={ 'Signal1', '0', '8', 'BE', 'unsigned', 'Standard', '0', '1', '0', '-Inf', 'Inf' }
      settings: LibrarySourceBlock=c2000lib/Target Communication/CAN Pack  DataFormat=raw data
  Constant22 : Constant  Value=10  OutDataTypeStr=uint8
  Constant23 : Constant  Value=0  OutDataTypeStr=uint8
  Constant24 : Constant  Value=hex2dec('0x0F')  OutDataTypeStr=uint8
  Mux4 : Mux  Inputs=3
  eCAN Transmit3 : c280xlib/CAN Transmit  chipFamily=C280x  useModule=CAN_A  mailboxNo=0  messageID=hex2dec('0x201')  messageType=Standard (11-bit identifier)  enableBlockingMode=on  postInterrupt=off  interruptLine=0
  wires:
  Mux4/1 -> CAN Pack/1
  CAN Pack/1 -> eCAN Transmit3/1
  Constant22/1 -> Mux4/3
  Constant23/1 -> Mux4/2
  Constant24/1 -> Mux4/1

== system HRXDUAL_Delay/Read position2/Subsystem5/Enable Motor2 (PDO)3 ==
  function : TriggerPort  TriggerType=function-call  VariantControl=(inherit)
  CAN Pack : canmsglib/CAN Pack  MsgList=(none)  MsgName=CAN Msg  MsgIDType=Standard (11-bit identifier)  MsgIdentifier=hex2dec('0x202')  MsgLength=3  Remote=off  ApplyMinMax=off  BusOutput=off  SignalInfo={ 'Signal1', '0', '8', 'BE', 'unsigned', 'Standard', '0', '1', '0', '-Inf', 'Inf' }
      settings: LibrarySourceBlock=c2000lib/Target Communication/CAN Pack  DataFormat=raw data
  Constant22 : Constant  Value=10  OutDataTypeStr=uint8
  Constant23 : Constant  Value=0  OutDataTypeStr=uint8
  Constant24 : Constant  Value=hex2dec('0x0F')  OutDataTypeStr=uint8
  Mux4 : Mux  Inputs=3
  eCAN Transmit3 : c280xlib/CAN Transmit  chipFamily=C280x  useModule=CAN_A  mailboxNo=0  messageID=hex2dec('0x202')  messageType=Standard (11-bit identifier)  enableBlockingMode=on  postInterrupt=off  interruptLine=0
  wires:
  Mux4/1 -> CAN Pack/1
  CAN Pack/1 -> eCAN Transmit3/1
  Constant22/1 -> Mux4/3
  Constant23/1 -> Mux4/2
  Constant24/1 -> Mux4/1

== system HRXDUAL_Delay/Read position2/Subsystem5/Set Motor Ready (PDO) ==
  function : TriggerPort  TriggerType=function-call  VariantControl=(inherit)
  CAN Pack : canmsglib/CAN Pack  MsgList=(none)  MsgName=CAN Msg  MsgIDType=Standard (11-bit identifier)  MsgIdentifier=hex2dec('0x202')  MsgLength=3  Remote=off  ApplyMinMax=off  BusOutput=off  SignalInfo={ 'Signal1', '0', '8', 'BE', 'unsigned', 'Standard', '0', '1', '0', '-Inf', 'Inf' }
      settings: LibrarySourceBlock=c2000lib/Target Communication/CAN Pack  DataFormat=raw data
  Constant22 : Constant  Value=10  OutDataTypeStr=uint8
  Constant23 : Constant  Value=0  OutDataTypeStr=uint8
  Constant24 : Constant  Value=hex2dec('0x06')  OutDataTypeStr=uint8
  Mux4 : Mux  Inputs=3
  eCAN Transmit3 : c280xlib/CAN Transmit  chipFamily=C280x  useModule=CAN_A  mailboxNo=1  messageID=hex2dec('0x202')  messageType=Standard (11-bit identifier)  enableBlockingMode=on  postInterrupt=off  interruptLine=0
  wires:
  Constant24/1 -> Mux4/1
  Constant23/1 -> Mux4/2
  Constant22/1 -> Mux4/3
  Mux4/1 -> CAN Pack/1
  CAN Pack/1 -> eCAN Transmit3/1

== system HRXDUAL_Delay/Read position2/Subsystem5/Set Motor Ready (PDO)1 ==
  function : TriggerPort  TriggerType=function-call  VariantControl=(inherit)
  CAN Pack : canmsglib/CAN Pack  MsgList=(none)  MsgName=CAN Msg  MsgIDType=Standard (11-bit identifier)  MsgIdentifier=hex2dec('0x201')  MsgLength=3  Remote=off  ApplyMinMax=off  BusOutput=off  SignalInfo={ 'Signal1', '0', '8', 'BE', 'unsigned', 'Standard', '0', '1', '0', '-Inf', 'Inf' }
      settings: LibrarySourceBlock=c2000lib/Target Communication/CAN Pack  DataFormat=raw data
  Constant22 : Constant  Value=10  OutDataTypeStr=uint8
  Constant23 : Constant  Value=0  OutDataTypeStr=uint8
  Constant24 : Constant  Value=hex2dec('0x06')  OutDataTypeStr=uint8
  Mux4 : Mux  Inputs=3
  eCAN Transmit3 : c280xlib/CAN Transmit  chipFamily=C280x  useModule=CAN_A  mailboxNo=0  messageID=hex2dec('0x201')  messageType=Standard (11-bit identifier)  enableBlockingMode=on  postInterrupt=off  interruptLine=0
  wires:
  Constant24/1 -> Mux4/1
  Constant23/1 -> Mux4/2
  Constant22/1 -> Mux4/3
  Mux4/1 -> CAN Pack/1
  CAN Pack/1 -> eCAN Transmit3/1

== system HRXDUAL_Delay/Read position2/Subsystem5/Set Motor2 Ready (PDO)2 ==
  function : TriggerPort  TriggerType=function-call  VariantControl=(inherit)
  CAN Pack : canmsglib/CAN Pack  MsgList=(none)  MsgName=CAN Msg  MsgIDType=Standard (11-bit identifier)  MsgIdentifier=hex2dec('0x202')  MsgLength=3  Remote=off  ApplyMinMax=off  BusOutput=off  SignalInfo={ 'Signal1', '0', '8', 'BE', 'unsigned', 'Standard', '0', '1', '0', '-Inf', 'Inf' }
      settings: LibrarySourceBlock=c2000lib/Target Communication/CAN Pack  DataFormat=raw data
  Constant22 : Constant  Value=10  OutDataTypeStr=uint8
  Constant23 : Constant  Value=0  OutDataTypeStr=uint8
  Constant24 : Constant  Value=hex2dec('0x06')  OutDataTypeStr=uint8
  Mux4 : Mux  Inputs=3
  eCAN Transmit3 : c280xlib/CAN Transmit  chipFamily=C280x  useModule=CAN_A  mailboxNo=0  messageID=hex2dec('0x202')  messageType=Standard (11-bit identifier)  enableBlockingMode=on  postInterrupt=off  interruptLine=0
  wires:
  Constant24/1 -> Mux4/1
  Constant23/1 -> Mux4/2
  Constant22/1 -> Mux4/3
  Mux4/1 -> CAN Pack/1
  CAN Pack/1 -> eCAN Transmit3/1

== system HRXDUAL_Delay/Read position2/Subsystem5/Set Torque Mode of Operation (PDO) ==
  function : TriggerPort  TriggerType=function-call  VariantControl=(inherit)
  CAN Pack : canmsglib/CAN Pack  MsgList=(none)  MsgName=CAN Msg  MsgIDType=Standard (11-bit identifier)  MsgIdentifier=hex2dec('0x202')  MsgLength=3  Remote=off  ApplyMinMax=off  BusOutput=off  SignalInfo={ 'Signal1', '0', '8', 'BE', 'unsigned', 'Standard', '0', '1', '0', '-Inf', 'Inf' }
      settings: LibrarySourceBlock=c2000lib/Target Communication/CAN Pack  DataFormat=raw data
  Constant22 : Constant  Value=10  OutDataTypeStr=uint8
  Constant23 : Constant  Value=0  OutDataTypeStr=uint8
  Constant24 : Constant  Value=0  OutDataTypeStr=uint8
  Mux4 : Mux  Inputs=3
  eCAN Transmit3 : c280xlib/CAN Transmit  chipFamily=C280x  useModule=CAN_A  mailboxNo=1  messageID=hex2dec('0x202')  messageType=Standard (11-bit identifier)  enableBlockingMode=on  postInterrupt=off  interruptLine=0
  wires:
  Mux4/1 -> CAN Pack/1
  CAN Pack/1 -> eCAN Transmit3/1
  Constant24/1 -> Mux4/1
  Constant22/1 -> Mux4/3
  Constant23/1 -> Mux4/2

== system HRXDUAL_Delay/Read position2/Subsystem5/Set Torque Mode of Operation (PDO)1 ==
  function : TriggerPort  TriggerType=function-call  VariantControl=(inherit)
  CAN Pack : canmsglib/CAN Pack  MsgList=(none)  MsgName=CAN Msg  MsgIDType=Standard (11-bit identifier)  MsgIdentifier=hex2dec('0x201')  MsgLength=3  Remote=off  ApplyMinMax=off  BusOutput=off  SignalInfo={ 'Signal1', '0', '8', 'BE', 'unsigned', 'Standard', '0', '1', '0', '-Inf', 'Inf' }
      settings: LibrarySourceBlock=c2000lib/Target Communication/CAN Pack  DataFormat=raw data
  Constant22 : Constant  Value=10  OutDataTypeStr=uint8
  Constant23 : Constant  Value=0  OutDataTypeStr=uint8
  Constant24 : Constant  Value=0  OutDataTypeStr=uint8
  Mux4 : Mux  Inputs=3
  eCAN Transmit3 : c280xlib/CAN Transmit  chipFamily=C280x  useModule=CAN_A  mailboxNo=0  messageID=hex2dec('0x201')  messageType=Standard (11-bit identifier)  enableBlockingMode=on  postInterrupt=off  interruptLine=0
  wires:
  Mux4/1 -> CAN Pack/1
  CAN Pack/1 -> eCAN Transmit3/1
  Constant24/1 -> Mux4/1
  Constant22/1 -> Mux4/3
  Constant23/1 -> Mux4/2

== system HRXDUAL_Delay/Read position2/Subsystem5/Set Torque Mode of Operation (PDO)2 ==
  function : TriggerPort  TriggerType=function-call  VariantControl=(inherit)
  CAN Pack : canmsglib/CAN Pack  MsgList=(none)  MsgName=CAN Msg  MsgIDType=Standard (11-bit identifier)  MsgIdentifier=hex2dec('0x202')  MsgLength=3  Remote=off  ApplyMinMax=off  BusOutput=off  SignalInfo={ 'Signal1', '0', '8', 'BE', 'unsigned', 'Standard', '0', '1', '0', '-Inf', 'Inf' }
      settings: LibrarySourceBlock=c2000lib/Target Communication/CAN Pack  DataFormat=raw data
  Constant22 : Constant  Value=10  OutDataTypeStr=uint8
  Constant23 : Constant  Value=0  OutDataTypeStr=uint8
  Constant24 : Constant  Value=0  OutDataTypeStr=uint8
  Mux4 : Mux  Inputs=3
  eCAN Transmit3 : c280xlib/CAN Transmit  chipFamily=C280x  useModule=CAN_A  mailboxNo=0  messageID=hex2dec('0x202')  messageType=Standard (11-bit identifier)  enableBlockingMode=on  postInterrupt=off  interruptLine=0
  wires:
  Mux4/1 -> CAN Pack/1
  CAN Pack/1 -> eCAN Transmit3/1
  Constant24/1 -> Mux4/1
  Constant22/1 -> Mux4/3
  Constant23/1 -> Mux4/2

== system HRXDUAL_Delay/Read position2/Subsystem5/Subsystem1 ==
  In1 : Inport
  function : TriggerPort  TriggerType=function-call  VariantControl=(inherit)
  CAN Pack : canmsglib/CAN Pack  MsgList=(none)  MsgName=CAN Msg  MsgIDType=Standard (11-bit identifier)  MsgIdentifier=0  MsgLength=2  Remote=off  ApplyMinMax=off  BusOutput=off  SignalInfo={ 'Signal1', '0', '8', 'BE', 'unsigned', 'Standard', '0', '1', '0', '-Inf', 'Inf' }
      settings: LibrarySourceBlock=c2000lib/Target Communication/CAN Pack  DataFormat=raw data
  eCAN Transmit3 : c280xlib/CAN Transmit  chipFamily=C280x  useModule=CAN_A  mailboxNo=0  messageID=0  messageType=Standard (11-bit identifier)  enableBlockingMode=on  postInterrupt=off  interruptLine=0
  wires:
  CAN Pack/1 -> eCAN Transmit3/1
  In1/1 -> CAN Pack/1

== system HRXDUAL_Delay/Read position2/Subsystem5/Subsystem4 ==
  In1 : Inport
  function : TriggerPort  TriggerType=function-call  VariantControl=(inherit)
  CAN Pack : canmsglib/CAN Pack  MsgList=(none)  MsgName=CAN Msg  MsgIDType=Standard (11-bit identifier)  MsgIdentifier=0  MsgLength=2  Remote=off  ApplyMinMax=off  BusOutput=off  SignalInfo={ 'Signal1', '0', '8', 'BE', 'unsigned', 'Standard', '0', '1', '0', '-Inf', 'Inf' }
      settings: LibrarySourceBlock=c2000lib/Target Communication/CAN Pack  DataFormat=raw data
  eCAN Transmit3 : c280xlib/CAN Transmit  chipFamily=C280x  useModule=CAN_A  mailboxNo=1  messageID=0  messageType=Standard (11-bit identifier)  enableBlockingMode=on  postInterrupt=off  interruptLine=0
  wires:
  CAN Pack/1 -> eCAN Transmit3/1
  In1/1 -> CAN Pack/1

== system HRXDUAL_Delay/Read position2/Subsystem5/Switch On Motor (PDO) ==
  function : TriggerPort  TriggerType=function-call  VariantControl=(inherit)
  CAN Pack : canmsglib/CAN Pack  MsgList=(none)  MsgName=CAN Msg  MsgIDType=Standard (11-bit identifier)  MsgIdentifier=hex2dec('0x202')  MsgLength=3  Remote=off  ApplyMinMax=off  BusOutput=off  SignalInfo={ 'Signal1', '0', '8', 'BE', 'unsigned', 'Standard', '0', '1', '0', '-Inf', 'Inf' }
      settings: LibrarySourceBlock=c2000lib/Target Communication/CAN Pack  DataFormat=raw data
  Constant22 : Constant  Value=10  OutDataTypeStr=uint8
  Constant23 : Constant  Value=0  OutDataTypeStr=uint8
  Constant24 : Constant  Value=hex2dec('0x07')  OutDataTypeStr=uint8
  Mux4 : Mux  Inputs=3
  eCAN Transmit3 : c280xlib/CAN Transmit  chipFamily=C280x  useModule=CAN_A  mailboxNo=1  messageID=hex2dec('0x202')  messageType=Standard (11-bit identifier)  enableBlockingMode=on  postInterrupt=off  interruptLine=0
  wires:
  Mux4/1 -> CAN Pack/1
  CAN Pack/1 -> eCAN Transmit3/1
  Constant22/1 -> Mux4/3
  Constant23/1 -> Mux4/2
  Constant24/1 -> Mux4/1

== system HRXDUAL_Delay/Read position2/Subsystem5/Switch On Motor (PDO)1 ==
  function : TriggerPort  TriggerType=function-call  VariantControl=(inherit)
  CAN Pack : canmsglib/CAN Pack  MsgList=(none)  MsgName=CAN Msg  MsgIDType=Standard (11-bit identifier)  MsgIdentifier=hex2dec('0x201')  MsgLength=3  Remote=off  ApplyMinMax=off  BusOutput=off  SignalInfo={ 'Signal1', '0', '8', 'BE', 'unsigned', 'Standard', '0', '1', '0', '-Inf', 'Inf' }
      settings: LibrarySourceBlock=c2000lib/Target Communication/CAN Pack  DataFormat=raw data
  Constant22 : Constant  Value=10  OutDataTypeStr=uint8
  Constant23 : Constant  Value=0  OutDataTypeStr=uint8
  Constant24 : Constant  Value=hex2dec('0x07')  OutDataTypeStr=uint8
  Mux4 : Mux  Inputs=3
  eCAN Transmit3 : c280xlib/CAN Transmit  chipFamily=C280x  useModule=CAN_A  mailboxNo=0  messageID=hex2dec('0x201')  messageType=Standard (11-bit identifier)  enableBlockingMode=on  postInterrupt=off  interruptLine=0
  wires:
  Mux4/1 -> CAN Pack/1
  CAN Pack/1 -> eCAN Transmit3/1
  Constant22/1 -> Mux4/3
  Constant23/1 -> Mux4/2
  Constant24/1 -> Mux4/1

== system HRXDUAL_Delay/Read position2/Subsystem5/Switch On Motor2 (PDO)2 ==
  function : TriggerPort  TriggerType=function-call  VariantControl=(inherit)
  CAN Pack : canmsglib/CAN Pack  MsgList=(none)  MsgName=CAN Msg  MsgIDType=Standard (11-bit identifier)  MsgIdentifier=hex2dec('0x202')  MsgLength=3  Remote=off  ApplyMinMax=off  BusOutput=off  SignalInfo={ 'Signal1', '0', '8', 'BE', 'unsigned', 'Standard', '0', '1', '0', '-Inf', 'Inf' }
      settings: LibrarySourceBlock=c2000lib/Target Communication/CAN Pack  DataFormat=raw data
  Constant22 : Constant  Value=10  OutDataTypeStr=uint8
  Constant23 : Constant  Value=0  OutDataTypeStr=uint8
  Constant24 : Constant  Value=hex2dec('0x07')  OutDataTypeStr=uint8
  Mux4 : Mux  Inputs=3
  eCAN Transmit3 : c280xlib/CAN Transmit  chipFamily=C280x  useModule=CAN_A  mailboxNo=0  messageID=hex2dec('0x202')  messageType=Standard (11-bit identifier)  enableBlockingMode=on  postInterrupt=off  interruptLine=0
  wires:
  Mux4/1 -> CAN Pack/1
  CAN Pack/1 -> eCAN Transmit3/1
  Constant22/1 -> Mux4/3
  Constant23/1 -> Mux4/2
  Constant24/1 -> Mux4/1

== system HRXDUAL_Delay/Read position2/Subsystem5/Delay 1ms/System Outputs ==

== system HRXDUAL_Delay/Read position2/Subsystem5/Delay 1ms1/System Outputs ==

== system HRXDUAL_Delay/Read position2/Subsystem5/Delay 1ms10/System Outputs ==

== system HRXDUAL_Delay/Read position2/Subsystem5/Delay 1ms11/System Outputs ==

== system HRXDUAL_Delay/Read position2/Subsystem5/Delay 1ms2/System Outputs ==

== system HRXDUAL_Delay/Read position2/Subsystem5/Delay 1ms3/System Outputs ==
